simulink model "test"  (R2022a)
settings: Solver=VariableStepAuto  StartTime=0.0  StopTime=10.0  RelTol=1e-3
libraries: slpidlib x1
settings Model: Creator=daixingze  LastModifiedBy=daixingze

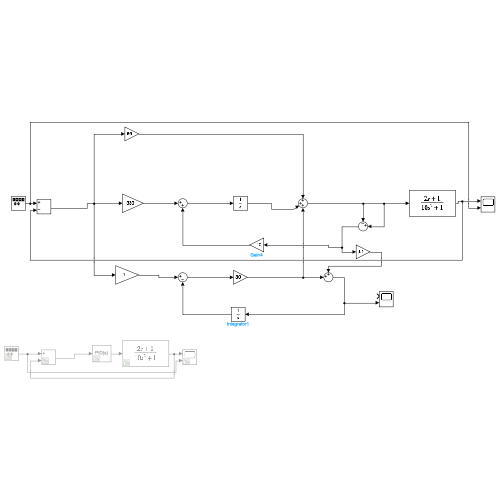
[thumbnail: Simulink's stored preview of the top-level diagram]
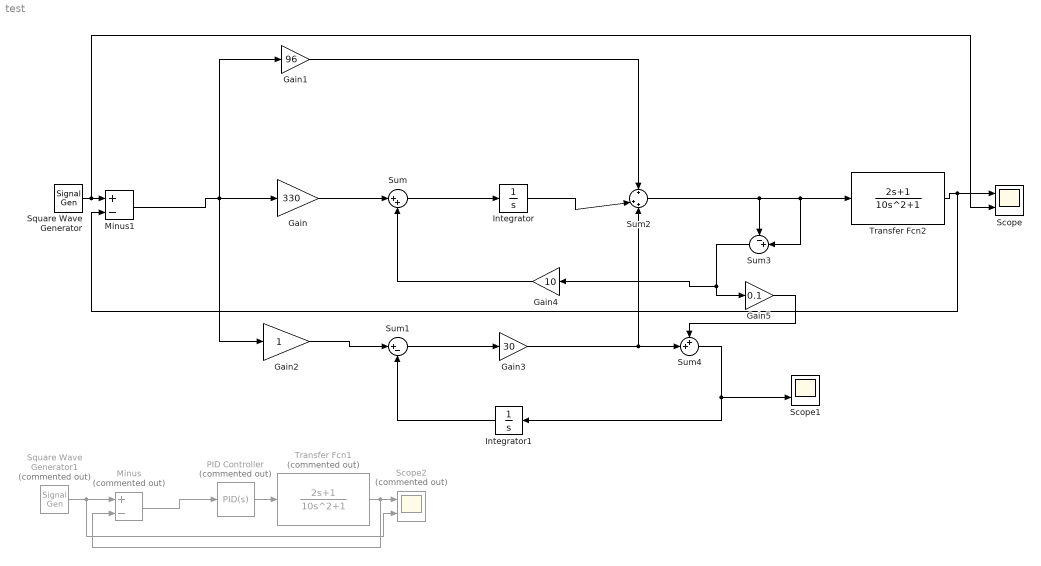
== system test ==
  Gain : Gain  Gain=330
  Gain1 : Gain  Gain=96
  Gain2 : Gain
  Gain3 : Gain  Gain=30
  Gain4 : Gain  Gain=10
  Gain5 : Gain  Gain=0.1
  Integrator : Integrator
  Integrator1 : Integrator
  Minus : Sum  Commented=on  Inputs=+-
  Minus1 : Sum  Inputs=+-
  PID Controller : slpidlib/PID Controller  Commented=on  Controller=PID  Form=Parallel  TimeDomain=Continuous-time  UseExternalTs=off  SampleTime=-1  IntegratorMethod=Forward Euler  FilterMethod=Forward Euler  ControllerParametersSource=internal  P=96.5243892669897  I=330.839138179468  UseKiTs=off  D=1.11685200842704  N=30.6984431842669  UseFilter=on  TunerSelectOption=Transfer Function Based (PID Tuner App)  InitialConditionSource=internal  InitialConditionForIntegrator=0  InitialConditionForFilter=0  DifferentiatorICPrevScaledInput=0  ExternalReset=none  TrackingMode=off  Kt=1  LimitOutput=off  SatLimitsSource=internal  UpperSaturationLimit=inf  LowerSaturationLimit=-inf  LinearizeAsGain=on  AntiWindupMode=none  Kb=1  POutMin=[]  POutMax=[]  IOutMin=[]  IOutMax=[]  DOutMin=[]  DOutMax=[]  NOutMin=[]  NOutMax=[]  SumOutMin=[]  SumOutMax=[]  SaturationOutMin=[]  SaturationOutMax=[]  PParamMin=[]  PParamMax=[]  IParamMin=[]  IParamMax=[]  DParamMin=[]  DParamMax=[]  NParamMin=[]  NParamMax=[]  KbParamMin=[]  KbParamMax=[]  KtParamMin=[]  KtParamMax=[]  KbOutMin=[]  KbOutMax=[]  KtOutMin=[]  KtOutMax=[]  IntegratorOutMin=[]  IntegratorOutMax=[]  FilterOutMin=[]  FilterOutMax=[]  SumI1OutMin=[]  SumI1OutMax=[]  SumI2OutMin=[]  SumI2OutMax=[]  SumI3OutMin=[]  SumI3OutMax=[]  SumI4OutMin=[]  SumI4OutMax=[]  SumDOutMin=[]  SumDOutMax=[]  DifferentiatorOutMin=[]  DifferentiatorOutMax=[]  FilterDiffOutCoefMin=[]  FilterDiffOutCoefMax=[]  ReciprocalOutMin=[]  ReciprocalOutMax=[]  SumDenOutMin=[]  SumDenOutMax=[]  SumNumOutMin=[]  SumNumOutMax=[]  DivideOutMin=[]  DivideOutMax=[]  UdiffTsProdOutMin=[]  UdiffTsProdOutMax=[]  NTsProdOutMin=[]  NTsProdOutMax=[]  UintegralTsProdOutMin=[]  UintegralTsProdOutMax=[]  UngainTsProdOutMin=[]  UngainTsProdOutMax=[]  ClampingZeroOutDataTypeStr=Inherit: Inherit via back propagation  ClampingZeroOutMin=[]  ClampingZeroOutMax=[]  FilterDenConstantOutDataTypeStr=Inherit: Inherit via back propagation  FilterDenConstantOutMin=[]  FilterDenConstantOutMax=[]  PCopyOutDataTypeStr=Inherit: Inherit via back propagation  PCopyOutMin=[]  PCopyOutMax=[]  NCopyOutDataTypeStr=Inherit: Inherit via back propagation  NCopyOutMin=[]  NCopyOutMax=[]  IntegratorContinuousStateAttributes=''  IntegratorStateMustResolveToSignalObject=off  IntegratorRTWStateStorageClass=Auto  FilterContinuousStateAttributes=''  FilterStateMustResolveToSignalObject=off  FilterRTWStateStorageClass=Auto  ParallelPVariant=InternalParameters  IdealPVariant=Disabled  IVariant=InternalParameters  DVariant=InternalParameters  IntegratorVariant=Continuous  SatVariant=Disabled  AWVariant=Passthrough  PCopyVariant=Disabled  TRVariant=Disabled  FdbkBlocksVariant=Forward  IdealPFdbkVariant=Disabled  SatFdbkVariant=Disabled  DerivativeFilterVariant=ContFilter  NVariant=InternalParameters  NCopyVariant=Disabled  FilterICVariant=InternalICsFilter  IntegratorICVariant=InternalICs  ExternalResetVariant=Disabled  TRSumVariant=Passthrough  SumFdbkVariant=Disabled  SumVariant=Sum_PID  TsampFilterVariant=InternalTs  TsampNgainVariant=Passthrough  TsampIntegralVariant=Passthrough  ExternalSaturationOutDataTypeStr=Inherit: Same as second input  aMode=0
  Scope : Scope  NumInputPorts=2
  Scope1 : Scope  NumInputPorts=2
  Scope2 : Scope  Commented=on  NumInputPorts=2
  Square Wave Generator : SignalGenerator  WaveForm=square  Units=rad/sec
  Square Wave Generator1 : SignalGenerator  Commented=on  WaveForm=square  Units=rad/sec
  Sum : Sum  Inputs=|++
  Sum1 : Sum  Inputs=|+-
  Sum2 : Sum  Inputs=+|++
  Sum3 : Sum  Inputs=-+|
  Sum4 : Sum  Inputs=++|
  Transfer Fcn1 : TransferFcn  Commented=on  Numerator=[2 1]  Denominator=[10 0 1]
  Transfer Fcn2 : TransferFcn  Numerator=[2 1]  Denominator=[10 0 1]
  wires:
  Gain/1 -> Sum/1
  Sum/1 -> Integrator/1
  Gain2/1 -> Sum1/1
  Sum1/1 -> Gain3/1
  Integrator/1 -> Sum2/2
  Gain1/1 -> Sum2/1
  Gain3/1 -> Sum4/2, Sum2/3
  Integrator1/1 -> Sum1/2
  Sum3/1 -> Gain5/1, Gain4/1
  Sum2/1 -> Transfer Fcn2/1, Sum3/2, Sum3/1
  Transfer Fcn2/1 -> Minus1/2, Scope/1
  PID Controller/1 -> Transfer Fcn1/1
  Transfer Fcn1/1 -> Minus/2, Scope2/1
  Square Wave Generator1/1 -> Scope2/2, Minus/1
  Minus/1 -> PID Controller/1
  Square Wave Generator/1 -> Scope/2, Minus1/1
  Minus1/1 -> Gain2/1, Gain1/1, Gain/1
  Sum4/1 -> Scope1/2, Integrator1/1
  Gain4/1 -> Sum/2
  Gain5/1 -> Sum4/1
